simulink model "walkingModel"  (R2013a)
settings: Solver=ode45  StartTime=0.0  StopTime=10  RelTol=1e-3
InitFcn:
  | walkingModel_params
values from neighbouring files (symbols this model uses):
  dx0 = 2    [walkingModel_params.m]
  dy0 = 0    [walkingModel_params.m]
  g = 9.81    [walkingModel_params.m]
  m = 70    [walkingModel_params.m]
  x0 = 0    [walkingModel_params.m]
  xF = sqrt(l^2 - y0^2)    [walkingModel_params.m]
  y0 = 0.9    [walkingModel_params.m]
libraries: simulink x1
settings Model: Creator=benshih  LastModifiedBy=benshih

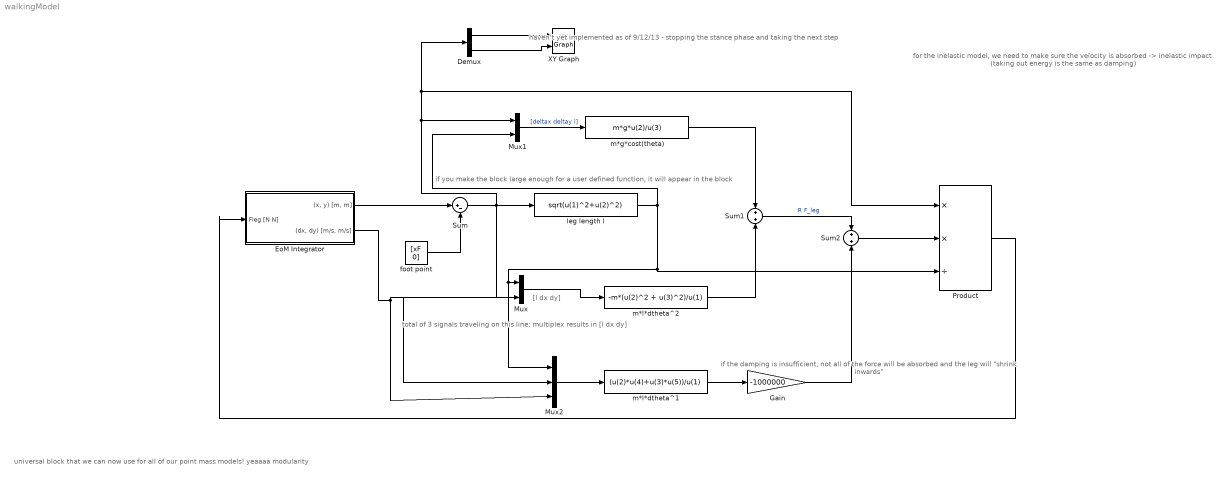
== system walkingModel ==
  note: if the damping is insufficient,
      | not all of the force will be absorbed
      | and the leg will "shrink inwards"
  note: haven't yet implemented as of 9/12/13 -
      | stopping the stance phase
      | and taking the next step
  note: for the inelastic model, we need
      | to make sure the
      | velocity is absorbed
      | -> inelastic impact
      | (taking out energy is the same as damping)
  note: [l dx dy]
  note: if you make the block large enough for a user defined function, it will appear in the block
  note: total of 3 signals traveling on this line: multiplex results in [l dx dy]
  note: universal block that we can now
      | use for all of our point mass models!
      | yeaaaa modularity
  Demux : Demux  Outputs=2
  "EoM Integrator " : Subsystem
  Gain : Gain  Gain=-1000000
  Mux : Mux  Inputs=2
  Mux1 : Mux  Inputs=2
  Mux2 : Mux  Inputs=3
  Product : Product  Inputs=**/
  Sum : Sum  Inputs=|+-
  Sum1 : Sum
  Sum2 : Sum
  XY Graph : simulink/Sinks/XY Graph  xmin=-1  xmax=1  ymin=0  ymax=1.1  st=0.01
  foot point : Constant  Value=[xF 0]
  leg length l : Fcn  Expr=sqrt(u(1)^2+u(2)^2)
  m*g*cost(theta) : Fcn  Expr=m*g*u(2)/u(3)
  m*l*dtheta^1 : Fcn  Expr=(u(2)*u(4)+u(3)*u(5))/u(1)
  m*l*dtheta^2 : Fcn  Expr=-m*(u(2)^2 + u(3)^2)/u(1)
  wires:
  foot point/1 -> Sum/2
  "EoM Integrator "/1("(x, y) [m, m]") -> Sum/1
  Sum/1 -> Mux2/2, Product/1, Demux/1, Mux1/1, leg length l/1
  Mux/1 -> m*l*dtheta^2/1
  "EoM Integrator "/2("(dx, dy) [m/s, m/s]") -> Mux2/3, Mux/2
  leg length l/1 -> Product/3, Mux2/1, Mux/1, Mux1/2
  Mux1/1 -> m*g*cost(theta)/1  "[deltax deltay l]"
  m*g*cost(theta)/1 -> Sum1/1
  m*l*dtheta^2/1 -> Sum1/2
  Sum1/1 -> Sum2/1  "R F_leg"
  Mux2/1 -> m*l*dtheta^1/1
  m*l*dtheta^1/1 -> Gain/1
  Gain/1 -> Sum2/2
  Sum2/1 -> Product/2
  Product/1 -> "EoM Integrator "/1("Fleg [N N] ")
  Demux/1 -> XY Graph/1
  Demux/2 -> XY Graph/2

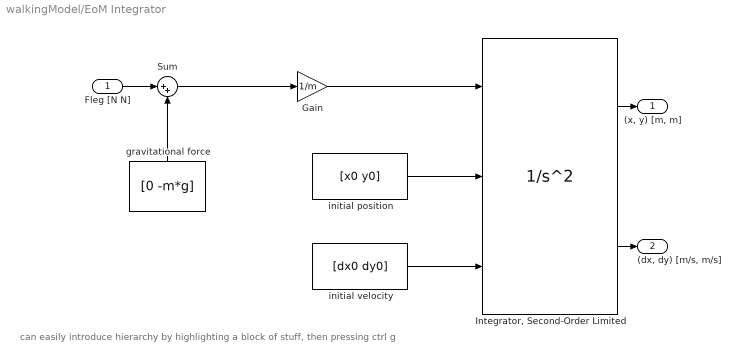
== system walkingModel/EoM Integrator  ==
  note: can easily introduce hierarchy by highlighting a block of stuff, then pressing ctrl g
  "Fleg [N N] " : Inport
  Gain : Gain  Gain=1/m
  "Integrator, Second-Order Limited" : SecondOrderIntegrator  ICSourceX=external  UpperLimitX=1  LowerLimitX=0  ICSourceDXDT=external
  Sum : Sum  Inputs=|++
  "gravitational force " : Constant  Value=[0 -m*g]
  "initial position " : Constant  Value=[x0 y0]
  initial velocity : Constant  Value=[dx0 dy0]
  "(x, y) [m, m]" : Outport
  "(dx, dy) [m/s, m/s]" : Outport  Port=2
  wires:
  "Integrator, Second-Order Limited"/2 -> "(dx, dy) [m/s, m/s]"/1
  Sum/1 -> Gain/1
  "initial position "/1 -> "Integrator, Second-Order Limited"/2
  "Integrator, Second-Order Limited"/1 -> "(x, y) [m, m]"/1
  "gravitational force "/1 -> Sum/2
  initial velocity/1 -> "Integrator, Second-Order Limited"/3
  "Fleg [N N] "/1 -> Sum/1
  Gain/1 -> "Integrator, Second-Order Limited"/1
